simulink library "SoftclipperBtc"  (R2022b)
settings: Solver=VariableStepAuto  StartTime=0.0  StopTime=10.0  RelTol=1e-3
undefined symbols (not defined in the file or in its folder): Column
libraries: TuneVar x6, TOP x6, FeaturePath x1, HandyTextFile x1
settings Model: Creator=db1045444  LastModifiedBy=kl13806
settings SolverCC: AlgebraicLoopSolver=TrustRegion
settings DebuggingCC: UnconnectedInputMsg=warning  UnconnectedOutputMsg=warning  UnconnectedLineMsg=warning  SFMachineParentedDataDiag=warning
settings ModelReferenceCC: EnableRefExpFcnMdlSchedulingChecks=on
settings RTWCC: DLArmComputeVersion=19.05

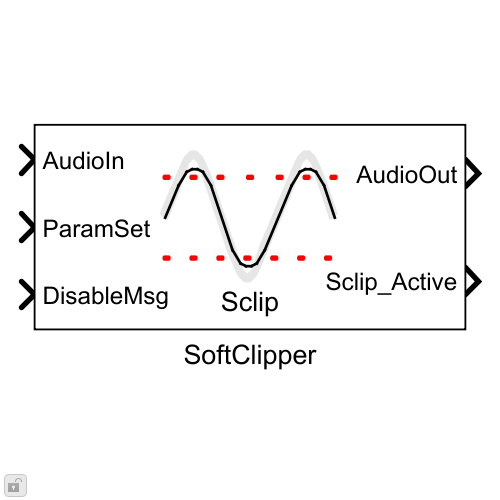
[thumbnail: Simulink's stored preview of the top-level diagram]
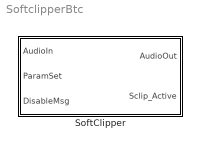
== system SoftclipperBtc ==
  SoftClipper : Subsystem  mask(Blocklib SoftClipper){Config=[], FeatureName=Sclip}
      mask prompts: Config "SoftClipperConfig"; FeatureName "Feature path name:"
      mask init:
      | blkh=gcbh;
      | Config=BTConfig.Assert(blkh,Config);
      | 
      | Config.Validate();
      | BTConfig.InitSetFeatureIfPresent(blkh,'FeatureName');
      mask Callback Config: BTConfig.CallbackHideIfPresent(gcbh,{'FeatureName'});
      mask TypeOptions FeatureName: FeaturePath/FeatureName
      mask Display:
      | [path,w,h] = IconSoftclipperMask();
      | 
      | % work in pixels since the icon does not scale
      | pos = get(gcbh,'position');
      | bw = pos(3) - pos(1);
      | bh = pos(4) - pos(2);
      | 
      | % Draw centered icon
      | xAdj = bw/2 - w/2;
      | yAdj = bh/2 - h/2 + 4;
      | for i=1:length(path)
      |     if (path(i).rgb(1) >= 0)
      |         patch(path(i).x+xAdj, path(i).y+yAdj, path(i).rgb);
      |     end
      |     if (path(i).stroke(1) >= 0)
      |         plot(path(i).x+xAdj, path(i).y+yAdj);
      |     end
      | end
      | 
      | % Display some text
      | text(bw/2, 4,FeatureName, ...
      |     'horizontalAlignment','center', ...
      |     'VerticalAlignment','bottom');

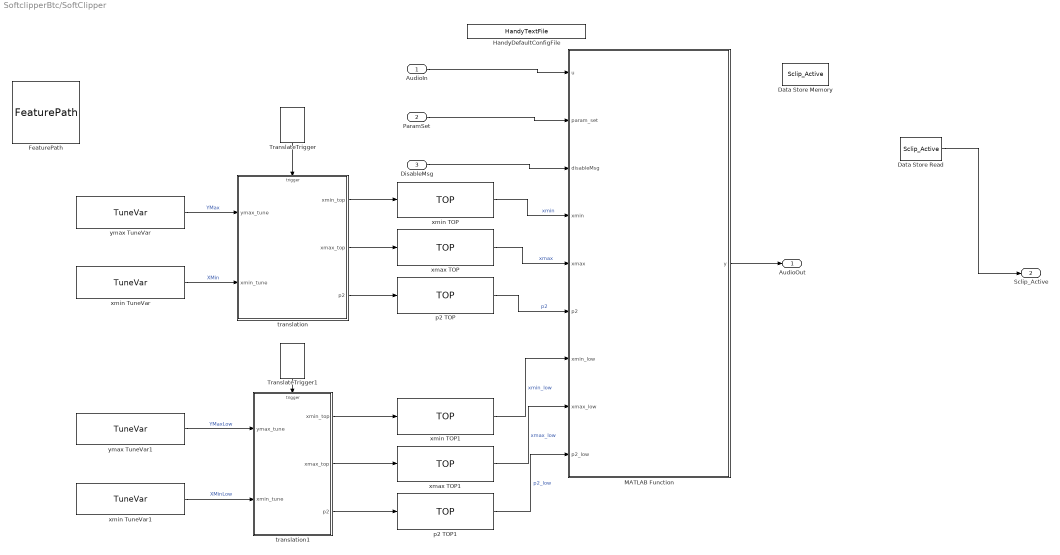
== system SoftclipperBtc/SoftClipper ==
  AudioIn : Inport
  ParamSet : Inport  Port=2
  DisableMsg : Inport  Port=3
  Data Store Memory : DataStoreMemory  DataStoreName=Sclip_Active  ShowAdditionalParam=off  OutDataTypeStr=uint32
  Data Store Read : DataStoreRead  DataStoreName=Sclip_Active  IndexOptions=Index vector (dialog)  Indices=1  OutputSizes=1
  FeaturePath : FeaturePath/FeaturePath  FeatureName=Sclip  IsGroup=off  GroupNumber=-1  IsModule=off  TriggerInit=[-80 -61 25 36]
      settings: SourceProductName=Bose Talaria
  HandyDefaultConfigFile : HandyTextFile/HandyTextFile  TemplateSource=Config  FileSuffix=Init  OpenDialogOnLoad=off  UseThisBlockName=off  AddGrandParentNamePrefix=off  TheDefaultText=|  ShowInLibBrowser=on
      | % $(FILENAME) Setup model parameters for each "Init" callback (e.g. update diagram)
      | sample_rate_in_hertz = 44100;
      | frame_size = 32;
      | sysin_channel_count = 2;
      settings: SourceProductName=Bose Talaria
  MATLAB Function : MATLAB Function  TreatAsAtomicUnit=on
  TranslateTrigger : TuneVar/TranslateTrigger  TriggerInit=[341 -20 379 35]
      settings: SourceProductName=Bose Talaria
  TranslateTrigger1 : TuneVar/TranslateTrigger  TriggerInit=[341 350 379 405]
      settings: SourceProductName=Bose Talaria
  p2 TOP : TOP/TOP  TriggerInit=[525 247 675 303]  TopName=p2  DataType=single  BankNumber=0  PreOverlay=false  PostOverlay=false  Role=Automatic
      settings: SourceProductName=Bose Talaria
  p2 TOP1 : TOP/TOP  TriggerInit=[525 587 675 643]  TopName=p2_low  DataType=single  BankNumber=0  PreOverlay=false  PostOverlay=false  Role=Automatic
      settings: SourceProductName=Bose Talaria
  translation : MATLAB Function  TreatAsAtomicUnit=on
  translation1 : MATLAB Function  TreatAsAtomicUnit=on
  xmax TOP : TOP/TOP  TriggerInit=[525 172 675 228]  TopName=xmax  DataType=single  BankNumber=0  PreOverlay=false  PostOverlay=false  Role=Automatic
      settings: SourceProductName=Bose Talaria
  xmax TOP1 : TOP/TOP  TriggerInit=[525 512 675 568]  TopName=xmax_low  DataType=single  BankNumber=0  PreOverlay=false  PostOverlay=false  Role=Automatic
      settings: SourceProductName=Bose Talaria
  xmin TOP : TOP/TOP  TriggerInit=[525 97 675 153]  TopName=xmin  DataType=single  BankNumber=0  PreOverlay=false  PostOverlay=false  Role=Automatic
      settings: SourceProductName=Bose Talaria
  xmin TOP1 : TOP/TOP  TriggerInit=[525 437 675 493]  TopName=xmin_low  DataType=single  BankNumber=0  PreOverlay=false  PostOverlay=false  Role=Automatic
      settings: SourceProductName=Bose Talaria
  xmin TuneVar : TuneVar/TuneVar  TuneName=XMin  SpecifyMaxSize=off  VariableDim=2 (Column)  MaxSize=[1 1]  TunabilityNumber=1  MinValue=[]  MaxValue=[]  TriggerInit=[20 230 190 280]  MaskValue=Config.DefaultXmin
      settings: SourceProductName=Bose Talaria
  xmin TuneVar1 : TuneVar/TuneVar  TuneName=XMinLow  SpecifyMaxSize=off  VariableDim=2 (Column)  MaxSize=[1 1]  TunabilityNumber=1  MinValue=[]  MaxValue=[]  TriggerInit=[20 570 190 620]  MaskValue=Config.DefaultXminLow
      settings: SourceProductName=Bose Talaria
  ymax TuneVar : TuneVar/TuneVar  TuneName=YMax  SpecifyMaxSize=off  VariableDim=2 (Column)  MaxSize=[1 1]  TunabilityNumber=1  MinValue=[]  MaxValue=[]  TriggerInit=[20 120 190 170]  MaskValue=Config.DefaultYmax
      settings: SourceProductName=Bose Talaria
  ymax TuneVar1 : TuneVar/TuneVar  TuneName=YMaxLow  SpecifyMaxSize=off  VariableDim=2 (Column)  MaxSize=[1 1]  TunabilityNumber=1  MinValue=[]  MaxValue=[]  TriggerInit=[20 460 190 510]  MaskValue=Config.DefaultYmaxLow
      settings: SourceProductName=Bose Talaria
  " AudioOut" : Outport  VectorParamsAs1DForOutWhenUnconnected=off
  Sclip_Active : Outport  Port=2
  wires:
  Data Store Read/1 -> Sclip_Active/1
  ParamSet/1 -> MATLAB Function/2(param_set)
  DisableMsg/1 -> MATLAB Function/3(disableMsg)
  AudioIn/1 -> MATLAB Function/1(u)
  MATLAB Function/1(y) -> " AudioOut"/1
  xmin TOP/1 -> MATLAB Function/4(xmin)  "xmin"
  xmax TOP/1 -> MATLAB Function/5(xmax)  "xmax"
  p2 TOP/1 -> MATLAB Function/6(p2)  "p2"
  translation/1(xmin_top) -> xmin TOP/1
  translation/2(xmax_top) -> xmax TOP/1
  translation/3(p2) -> p2 TOP/1
  ymax TuneVar/1 -> translation/1(ymax_tune)  "YMax"
  xmin TuneVar/1 -> translation/2(xmin_tune)  "XMin"
  TranslateTrigger/1 -> translation/Trigger
  TranslateTrigger1/1 -> translation1/Trigger
  ymax TuneVar1/1 -> translation1/1(ymax_tune)  "YMaxLow"
  xmin TuneVar1/1 -> translation1/2(xmin_tune)  "XMinLow"
  xmin TOP1/1 -> MATLAB Function/7(xmin_low)  "xmin_low"
  translation1/1(xmin_top) -> xmin TOP1/1
  xmax TOP1/1 -> MATLAB Function/8(xmax_low)  "xmax_low"
  p2 TOP1/1 -> MATLAB Function/9(p2_low)  "p2_low"
  translation1/3(p2) -> p2 TOP1/1
  translation1/2(xmax_top) -> xmax TOP1/1

== matlab function SoftclipperBtc/SoftClipper/translation ==
  data: ymax_tune input; xmin_top output; xmin_tune input; xmax_top output; p2 output
  events: trigger input FUNCTION_CALL_EVENT
function [xmin_top,xmax_top, p2] = fcn(ymax_tune, xmin_tune)

% Translates Ymax and Xmin to Xmax and Xmin

xmin_top = xmin_tune.Value;
xmax_top = 2 * ymax_tune.Value - xmin_top;

% p2 remains 0 unless below condition is met
% p2 is later used in the gain redux function 
p2 = 0;
if (xmax_top ~= xmin_top)
    p2 = 1 / (2 * (xmax_top - xmin_top));
end

== matlab function SoftclipperBtc/SoftClipper/MATLAB Function ==
  data: u input; param_set input; disableMsg input; y output; xmin input; xmax input; p2 input; xmin_low input; xmax_low input; p2_low input; Sclip_Active data_store_memory
function y = softclip(u, param_set, disableMsg, xmin, xmax, p2, xmin_low, xmax_low, p2_low)

% This is the main function for the Soft-Clipper
% It takes in audio, typically from the Limiter, and applies a gain
% reduction when appropriate. 
% It takes in two sets of tunable parameters.
% Each set represents values corresponding to a car that either stays on,
% or shuts off, when idling. 
y = coder.nullcopy(u);
[frame_size, channel_count] = size(u);

% Choose whether we are using the set of coefficients for a car that shuts
% off while idling, or not.
if (param_set == 1)
    xmin_param = xmin;
    xmax_param = xmax;
    p2_param = p2;
else
    xmin_param = xmin_low;
    xmax_param = xmax_low;
    p2_param = p2_low;
end

global Sclip_Active
Sclip_Active = uint32(0);
% If RTC Disable message is 1, do not perform soft-clipping
if (disableMsg)
    y(:) = u(:);
else
%     Loop over all channels
    for i = 1:channel_count
%         Loop over each sample of each channel
        for j = 1:frame_size
            x1 = abs( u(j,i) );
            x1 = min(x1, xmax_param);
            x2 = x1 - xmin_param;
            x2 = max(x2, single(0));
            x2 = x2 * x2;
            x2 = x2 * p2_param;
            x1 = x1 - x2;
            y(j,i) = copysignf(x1, u(j,i));
        end  
        if (max(abs(u(:,i)))> xmin_param)
            Sclip_Active = Sclip_Active + 2^(i-1);
        end
    end
end

== matlab function SoftclipperBtc/SoftClipper/translation1 ==
  data: xmin_top output; ymax_tune input; xmin_tune input; xmax_top output; p2 output
  events: trigger input FUNCTION_CALL_EVENT
function [xmin_top,xmax_top, p2] = fcn(ymax_tune, xmin_tune)

% Translates Ymax and Xmin to Xmax and Xmin

xmin_top = xmin_tune.Value;
xmax_top = 2 * ymax_tune.Value - xmin_top;

% p2 remains 0 unless below condition is met
% p2 is later used in the gain redux function 
p2 = 0;
if (xmax_top ~= xmin_top)
    p2 = 1 / (2 * (xmax_top - xmin_top));
end
